simulink model "cic_model"  (R2022b)
settings: Solver=ode45  StartTime=0.0  StopTime=Tsim  RelTol=1e-3  EnableMultiTasking=on
values from neighbouring files (symbols this model uses):
  fo = 5    [sim_cic_model.m]
  Fsig = 15    [sim_cic_model.m]
  fsL = 48    [sim_cic_model.m]
  h_comp_cic = round(h_comp_cic*2^16)*2^-16    [sim_cic_model.m]
  M = 1    [sim_cic_model.m]
  R = 2000    [sim_cic_model.m]
  switch_case = 2    [sim_cic_model.m]
libraries: dspsigops x2, dspsrcs4 x1
settings Model: Creator=jvalls  LastModifiedBy=SMORSUA
settings SolverCC: AlgebraicLoopSolver=TrustRegion
settings DataIOCC: LimitDataPoints=on  SaveFormat=Array  SignalLoggingSaveFormat=ModelDataLogs  ReturnWorkspaceOutputs=off
settings OptimizationCC: ExpressionDepthLimit=2147483647  LifeSpan=inf
settings DebuggingCC: UnderspecifiedInitializationDetection=Classic  MergeDetectMultiDrivingBlocksExec=none  SolverPrmCheckMsg=warning  ParameterPrecisionLossMsg=none  FcnCallInpInsideContextMsg=warning  UnconnectedInputMsg=warning  UnconnectedOutputMsg=warning  UnconnectedLineMsg=warning  StateNameClashWarn=warning  SFUnexpectedBacktrackingDiag=warning  SFNoUnconditionalDefaultTransitionDiag=warning  ArithmeticOperatorsInVariantConditions=warning
settings HardwareCC: ProdBitPerPointer=32  ProdBitPerSizeT=32  ProdBitPerPtrDiffT=32  ProdLargestAtomicFloat=None  ProdIntDivRoundTo=Undefined  ProdEndianess=Unspecified  ProdWordSize=32  ProdHWDeviceType=32-bit Generic
settings ModelReferenceCC: EnableRefExpFcnMdlSchedulingChecks=on  PropagateSignalLabelsOutOfModel=off
settings SFSimCC: SimUseLocalCustomCode=off  CustomCodeUndefinedFunction=UseInterfaceOnly
settings RTWCC: RTWUseLocalCustomCode=off
settings CodeAppCC: StateflowObjectComments=on
settings GRTTargetCC: TargetLangStandard=C89/C90 (ANSI)  CombineOutputUpdateFcns=off  GRTInterface=on
settings ConfigComp: CovMetricSettings=dw  CovSaveCumulativeToWorkspaceVar=on  CovSaveSingleToWorkspaceVar=on  CovExternalEMLEnable=off  CovSFcnEnable=off

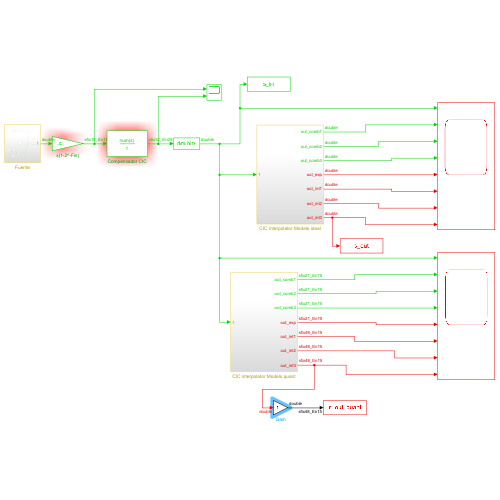
[thumbnail: Simulink's stored preview of the top-level diagram]
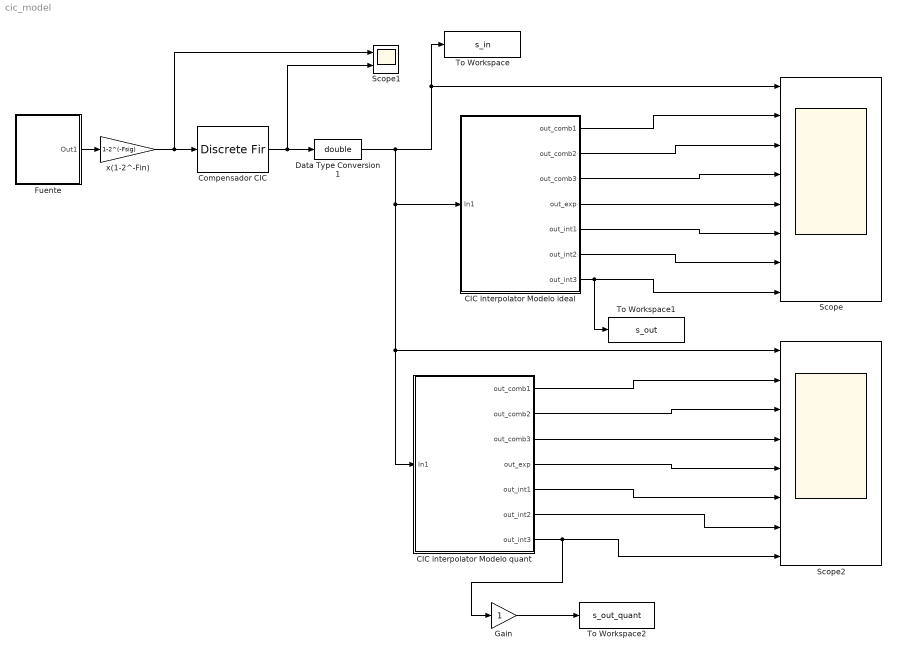
== system cic_model ==
  "CIC interpolator Modelo ideal " : Subsystem
  CIC interpolator Modelo quant : Subsystem
  Compensador CIC : DiscreteFir  Coefficients=h_comp_cic  InputProcessing=Columns as channels (frame based)
  Data Type Conversion1 : DataTypeConversion  OutDataTypeStr=double  SaturateOnIntegerOverflow=off  RndMeth=Floor
  Fuente : Subsystem
  Gain : Gain  OutDataTypeStr=double
  Scope : Scope  NumInputPorts=8
  Scope1 : Scope  NumInputPorts=2
  Scope2 : Scope  NumInputPorts=8
  To Workspace : ToWorkspace  VariableName=s_in  SampleTime=-1
      settings: Save2DSignal=2-D array (concatenate along first dimension)
  To Workspace1 : ToWorkspace  VariableName=s_out  SampleTime=-1
      settings: Save2DSignal=2-D array (concatenate along first dimension)
  To Workspace2 : ToWorkspace  VariableName=s_out_quant  SampleTime=-1
      settings: Save2DSignal=2-D array (concatenate along first dimension)
  x(1-2^-Fin) : Gain  Gain=1-2^(-Fsig)  OutDataTypeStr=fixdt(1,Wsig,Fsig)
  wires:
  Data Type Conversion1/1 -> Scope/1, To Workspace/1, Scope2/1, CIC interpolator Modelo quant/1(In1), "CIC interpolator Modelo ideal "/1(In1)
  Fuente/1(Out1) -> x(1-2^-Fin)/1
  x(1-2^-Fin)/1 -> Scope1/1, Compensador CIC/1
  Compensador CIC/1 -> Scope1/2, Data Type Conversion1/1
  "CIC interpolator Modelo ideal "/4(out_exp) -> Scope/5
  "CIC interpolator Modelo ideal "/3(out_comb3) -> Scope/4
  "CIC interpolator Modelo ideal "/5(out_int1) -> Scope/6
  "CIC interpolator Modelo ideal "/2(out_comb2) -> Scope/3
  "CIC interpolator Modelo ideal "/6(out_int2) -> Scope/7
  "CIC interpolator Modelo ideal "/1(out_comb1) -> Scope/2
  "CIC interpolator Modelo ideal "/7(out_int3) -> To Workspace1/1, Scope/8
  CIC interpolator Modelo quant/1(out_comb1) -> Scope2/2
  CIC interpolator Modelo quant/2(out_comb2) -> Scope2/3
  CIC interpolator Modelo quant/3(out_comb3) -> Scope2/4
  CIC interpolator Modelo quant/4(out_exp) -> Scope2/5
  CIC interpolator Modelo quant/5(out_int1) -> Scope2/6
  CIC interpolator Modelo quant/6(out_int2) -> Scope2/7
  CIC interpolator Modelo quant/7(out_int3) -> Gain/1, Scope2/8
  Gain/1 -> To Workspace2/1

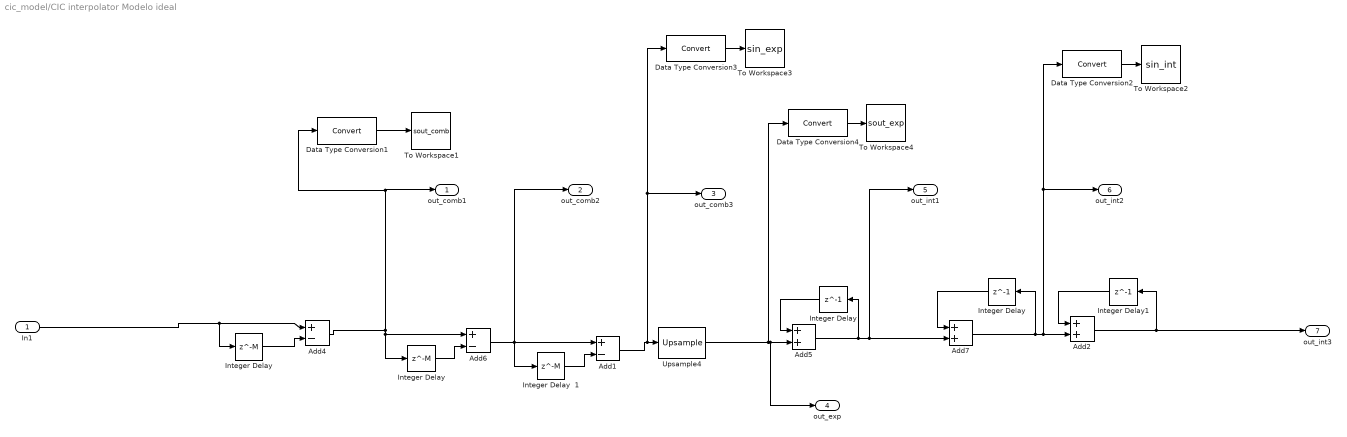
== system cic_model/CIC interpolator Modelo ideal  ==
  In1 : Inport
  " Integer Delay" : Delay  DelayLength=1
  " Integer Delay1" : Delay  DelayLength=1
  Add1 : Sum  Inputs=+-
  Add2 : Sum
  Add4 : Sum  Inputs=+-
  Add5 : Sum
  Add6 : Sum  Inputs=+-
  Add7 : Sum
  Data Type Conversion{1..4} (4 alike) : DataTypeConversion  SaturateOnIntegerOverflow=off  RndMeth=Floor
  "Integer Delay " : Delay  DelayLength=1
  "Integer Delay " : Delay  DelayLength=M
  "Integer Delay  " : Delay  DelayLength=M
  Integer Delay  1 : Delay  DelayLength=M
  To Workspace1 : ToWorkspace  VariableName=sout_comb  SampleTime=-1
      settings: Save2DSignal=2-D array (concatenate along first dimension)
  To Workspace2 : ToWorkspace  VariableName=sin_int  SampleTime=-1
      settings: Save2DSignal=2-D array (concatenate along first dimension)
  To Workspace3 : ToWorkspace  VariableName=sin_exp  SampleTime=-1
      settings: Save2DSignal=2-D array (concatenate along first dimension)
  To Workspace4 : ToWorkspace  VariableName=sout_exp  SampleTime=-1
      settings: Save2DSignal=2-D array (concatenate along first dimension)
  Upsample4 : dspsigops/Upsample  N=R  phase=0  InputProcessing=Columns as channels (frame based)  RateOptions=Allow multirate processing  ic=0  mode=Unused parameter value
  out_comb1 : Outport  VectorParamsAs1DForOutWhenUnconnected=off
  out_comb2 : Outport  Port=2  VectorParamsAs1DForOutWhenUnconnected=off
  out_comb3 : Outport  Port=3  VectorParamsAs1DForOutWhenUnconnected=off
  out_exp : Outport  Port=4  VectorParamsAs1DForOutWhenUnconnected=off
  out_int1 : Outport  Port=5  VectorParamsAs1DForOutWhenUnconnected=off
  out_int2 : Outport  Port=6  VectorParamsAs1DForOutWhenUnconnected=off
  out_int3 : Outport  Port=7  VectorParamsAs1DForOutWhenUnconnected=off
  wires:
  In1/1 -> "Integer Delay "/1, Add4/1
  " Integer Delay"/1 -> Add7/1
  "Integer Delay "/1 -> Add5/1
  "Integer Delay "/1 -> Add4/2
  "Integer Delay  "/1 -> Add6/2
  Integer Delay  1/1 -> Add1/2
  " Integer Delay1"/1 -> Add2/1
  Add6/1 -> out_comb2/1, Integer Delay  1/1, Add1/1
  Add4/1 -> "Integer Delay  "/1, Add6/1, Data Type Conversion1/1, out_comb1/1
  Add7/1 -> Data Type Conversion2/1, out_int2/1, Add2/2, " Integer Delay"/1
  Data Type Conversion1/1 -> To Workspace1/1
  Add5/1 -> "Integer Delay "/1, Add7/2, out_int1/1
  Data Type Conversion2/1 -> To Workspace2/1
  Data Type Conversion3/1 -> To Workspace3/1
  Add1/1 -> Data Type Conversion3/1, out_comb3/1, Upsample4/1
  Data Type Conversion4/1 -> To Workspace4/1
  Upsample4/1 -> Data Type Conversion4/1, out_exp/1, Add5/2
  Add2/1 -> out_int3/1, " Integer Delay1"/1

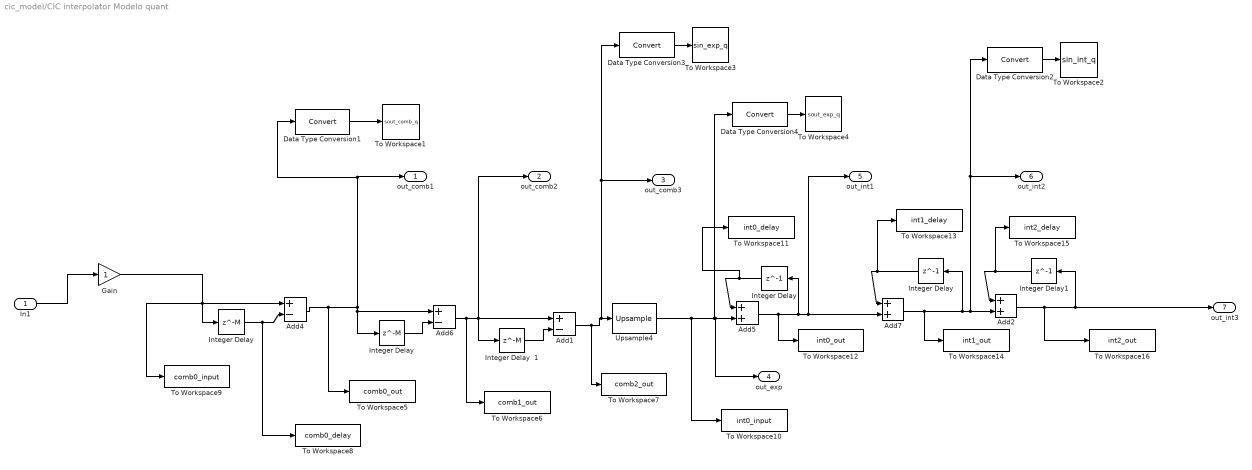
== system cic_model/CIC interpolator Modelo quant ==
  In1 : Inport
  " Integer Delay" : Delay  DelayLength=1
  " Integer Delay1" : Delay  DelayLength=1
  Add1 : Sum  Inputs=+-  OutDataTypeStr=fixdt(1,Wcomb,Fcomb)
  Add2 : Sum  OutDataTypeStr=fixdt(1,Wint,Fint)
  Add4 : Sum  Inputs=+-  OutDataTypeStr=fixdt(1,Wcomb,Fcomb)
  Add5 : Sum  OutDataTypeStr=fixdt(1,Wint,Fint)
  Add6 : Sum  Inputs=+-  OutDataTypeStr=fixdt(1,Wcomb,Fcomb)
  Add7 : Sum  OutDataTypeStr=fixdt(1,Wint,Fint)
  Data Type Conversion{1..4} (4 alike) : DataTypeConversion  SaturateOnIntegerOverflow=off  RndMeth=Floor
  Gain : Gain  OutDataTypeStr=fixdt(1,21,15)
  "Integer Delay " : Delay  DelayLength=1
  "Integer Delay " : Delay  DelayLength=M
  "Integer Delay  " : Delay  DelayLength=M
  Integer Delay  1 : Delay  DelayLength=M
  To Workspace1 : ToWorkspace  VariableName=sout_comb_q  SampleTime=-1
      settings: Save2DSignal=2-D array (concatenate along first dimension)
  To Workspace10 : ToWorkspace  VariableName=int0_input  SampleTime=-1
      settings: Save2DSignal=2-D array (concatenate along first dimension)
  To Workspace11 : ToWorkspace  VariableName=int0_delay  SampleTime=-1
      settings: Save2DSignal=2-D array (concatenate along first dimension)
  To Workspace12 : ToWorkspace  VariableName=int0_out  SampleTime=-1
      settings: Save2DSignal=2-D array (concatenate along first dimension)
  To Workspace13 : ToWorkspace  VariableName=int1_delay  SampleTime=-1
      settings: Save2DSignal=2-D array (concatenate along first dimension)
  To Workspace14 : ToWorkspace  VariableName=int1_out  SampleTime=-1
      settings: Save2DSignal=2-D array (concatenate along first dimension)
  To Workspace15 : ToWorkspace  VariableName=int2_delay  SampleTime=-1
      settings: Save2DSignal=2-D array (concatenate along first dimension)
  To Workspace16 : ToWorkspace  VariableName=int2_out  SampleTime=-1
      settings: Save2DSignal=2-D array (concatenate along first dimension)
  To Workspace2 : ToWorkspace  VariableName=sin_int_q  SampleTime=-1
      settings: Save2DSignal=2-D array (concatenate along first dimension)
  To Workspace3 : ToWorkspace  VariableName=sin_exp_q  SampleTime=-1
      settings: Save2DSignal=2-D array (concatenate along first dimension)
  To Workspace4 : ToWorkspace  VariableName=sout_exp_q  SampleTime=-1
      settings: Save2DSignal=2-D array (concatenate along first dimension)
  To Workspace5 : ToWorkspace  VariableName=comb0_out  SampleTime=-1
      settings: Save2DSignal=2-D array (concatenate along first dimension)
  To Workspace6 : ToWorkspace  VariableName=comb1_out  SampleTime=-1
      settings: Save2DSignal=2-D array (concatenate along first dimension)
  To Workspace7 : ToWorkspace  VariableName=comb2_out  SampleTime=-1
      settings: Save2DSignal=2-D array (concatenate along first dimension)
  To Workspace8 : ToWorkspace  VariableName=comb0_delay  SampleTime=-1
      settings: Save2DSignal=2-D array (concatenate along first dimension)
  To Workspace9 : ToWorkspace  VariableName=comb0_input  SampleTime=-1
      settings: Save2DSignal=2-D array (concatenate along first dimension)
  Upsample4 : dspsigops/Upsample  N=R  phase=0  InputProcessing=Columns as channels (frame based)  RateOptions=Allow multirate processing  ic=0  mode=Unused parameter value
  out_comb1 : Outport  VectorParamsAs1DForOutWhenUnconnected=off
  out_comb2 : Outport  Port=2  VectorParamsAs1DForOutWhenUnconnected=off
  out_comb3 : Outport  Port=3  VectorParamsAs1DForOutWhenUnconnected=off
  out_exp : Outport  Port=4  VectorParamsAs1DForOutWhenUnconnected=off
  out_int1 : Outport  Port=5  VectorParamsAs1DForOutWhenUnconnected=off
  out_int2 : Outport  Port=6  VectorParamsAs1DForOutWhenUnconnected=off
  out_int3 : Outport  Port=7  VectorParamsAs1DForOutWhenUnconnected=off
  wires:
  " Integer Delay"/1 -> To Workspace13/1, Add7/1
  "Integer Delay "/1 -> To Workspace11/1, Add5/1
  "Integer Delay "/1 -> To Workspace8/1, Add4/2
  "Integer Delay  "/1 -> Add6/2
  Integer Delay  1/1 -> Add1/2
  " Integer Delay1"/1 -> To Workspace15/1, Add2/1
  Add6/1 -> To Workspace6/1, out_comb2/1, Integer Delay  1/1, Add1/1
  Add4/1 -> To Workspace5/1, "Integer Delay  "/1, Add6/1, Data Type Conversion1/1, out_comb1/1
  Add7/1 -> To Workspace14/1, Data Type Conversion2/1, out_int2/1, Add2/2, " Integer Delay"/1
  Data Type Conversion1/1 -> To Workspace1/1
  Add5/1 -> To Workspace12/1, "Integer Delay "/1, Add7/2, out_int1/1
  Data Type Conversion2/1 -> To Workspace2/1
  Data Type Conversion3/1 -> To Workspace3/1
  Add1/1 -> To Workspace7/1, Data Type Conversion3/1, out_comb3/1, Upsample4/1
  Data Type Conversion4/1 -> To Workspace4/1
  Add2/1 -> To Workspace16/1, out_int3/1, " Integer Delay1"/1
  In1/1 -> Gain/1
  Gain/1 -> "Integer Delay "/1, Add4/1, To Workspace9/1
  Upsample4/1 -> To Workspace10/1, Data Type Conversion4/1, out_exp/1, Add5/2

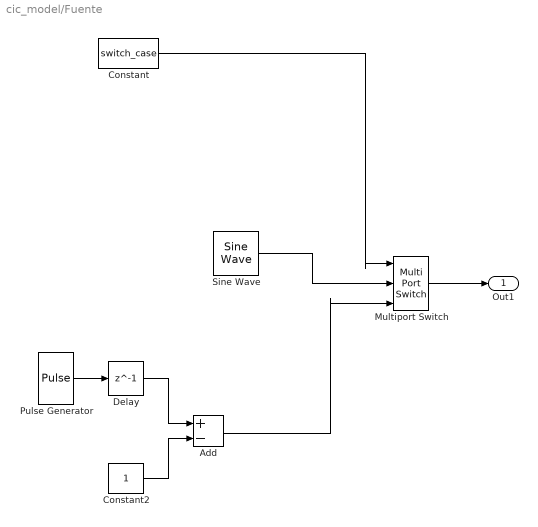
== system cic_model/Fuente ==
  Add : Sum  Inputs=+-
  Constant : Constant  Value=switch_case
  Constant2 : Constant
  Delay : Delay  DelayLength=1  InitialCondition=0  SampleTime=1/(fsL*1000)
  Multiport Switch : MultiPortSwitch  Inputs=2  SaturateOnIntegerOverflow=off  InputSameDT=off
  Pulse Generator : DiscretePulseGenerator  PulseType=Time based  Amplitude=2  Period=1/(fo*1000)  PulseWidth=50  SampleTime=1/(fsL*1000)
  Sine Wave : dspsrcs4/Sine Wave  Amplitude=1  Frequency=fo*1000  Phase=0  SampleMode=Discrete  OutComplex=Real  CompMethod=Trigonometric fcn  TableSize=Speed  SampleTime=1/(fsL*1000)  SamplesPerFrame=1  ResetState=Restart at time zero  OutputFrames=on  dataType=double  wordLen=16  udDataType=sfix(16)  fracBitsMode=User-defined  numFracBits=15  OutDataTypeStr=double  LastOutDataTypeStr=double
  Out1 : Outport  VectorParamsAs1DForOutWhenUnconnected=off
  wires:
  Multiport Switch/1 -> Out1/1
  Constant2/1 -> Add/2
  Delay/1 -> Add/1
  Pulse Generator/1 -> Delay/1
  Constant/1 -> Multiport Switch/1
  Sine Wave/1 -> Multiport Switch/2
  Add/1 -> Multiport Switch/3
